simulink model "SP_CV3S"  (R2025b)
settings: Solver=VariableStepAuto  StartTime=0.0  StopTime=1200  RelTol=1e-3
values from neighbouring files (symbols this model uses):
  g = 9.81    [SP_CV3.m]
  mu = 0.62    [SP_CV3.m]
  Q10 = 0.01942    [SP_CV3.m]
  S1 = 1    [SP_CV3.m]
  S10 = 100 * 1e-4    (= 0.01)    [SP_CV3.m]
  S2 = 1    [SP_CV3.m]
  S20 = 100 * 1e-4    (= 0.01)    [SP_CV3.m]
settings Model: Creator=jakub  LastModifiedBy=jakub

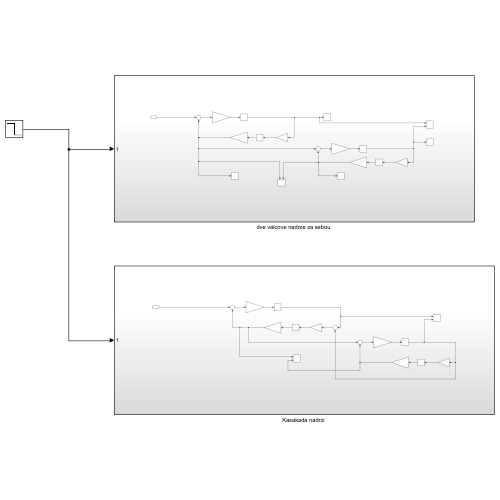
[thumbnail: Simulink's stored preview of the top-level diagram]
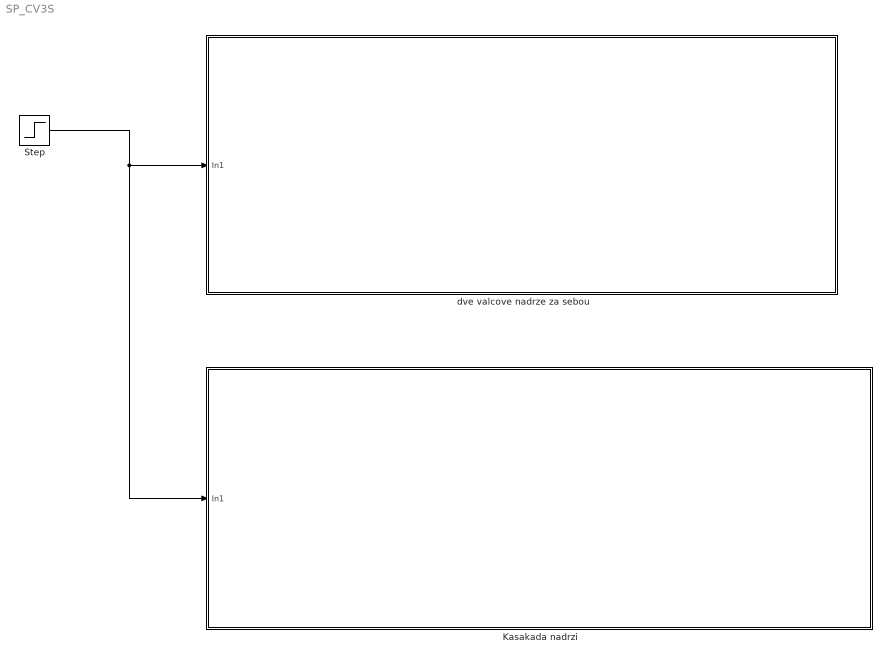
== system SP_CV3S ==
  "Kasakada nadrzi " : Subsystem
  Step : Step  Time=700  Before=Q10  After=Q10/2  SampleTime=0
  "dve valcove nadrze za sebou " : Subsystem
  wires:
  Step/1 -> "Kasakada nadrzi "/1(In1), "dve valcove nadrze za sebou "/1(In1)

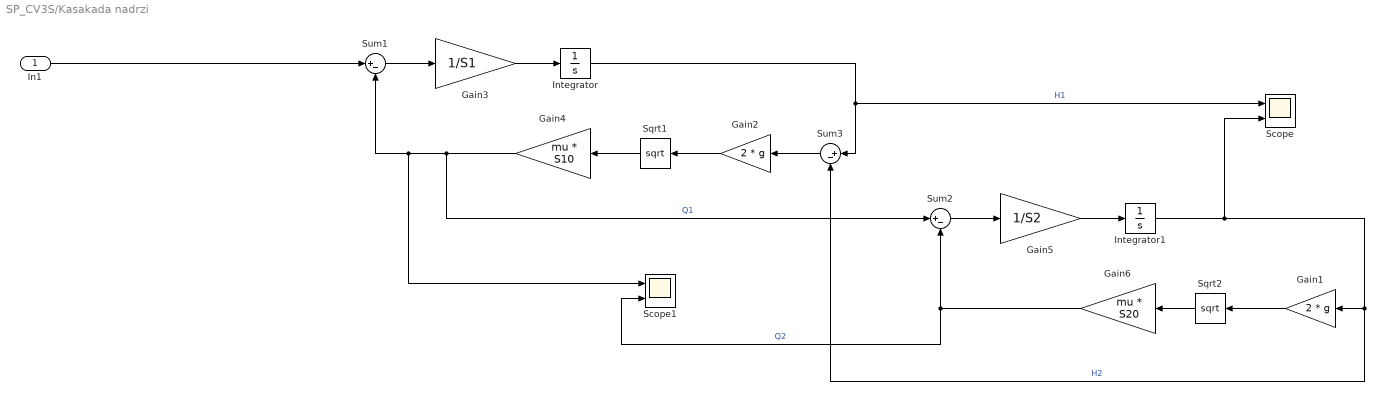
== system SP_CV3S/Kasakada nadrzi  ==
  In1 : Inport
  Gain1 : Gain  Gain=2 * g
  Gain2 : Gain  Gain=2 * g
  Gain3 : Gain  Gain=1/S1
  Gain4 : Gain  Gain=mu * S10
  Gain5 : Gain  Gain=1/S2
  Gain6 : Gain  Gain=mu * S20
  Integrator : Integrator
  Integrator1 : Integrator
  Scope : Scope  NumInputPorts=2
      settings: ActiveDisplayYMinimum=-0.12453477348635439  ActiveDisplayYMaximum=1.1208129613771898  DataLoggingVariableName=ScopeData6
  Scope1 : Scope  NumInputPorts=2
      settings: ActiveDisplayYMinimum=-0.0024239470723240262  ActiveDisplayYMaximum=0.021815523650916241  DataLoggingVariableName=ScopeData7
  Sqrt1 : Sqrt
  Sqrt2 : Sqrt
  Sum1 : Sum  Inputs=|+-
  Sum2 : Sum  Inputs=|+-
  Sum3 : Sum  Inputs=|+-
  wires:
  Integrator1/1 -> Scope/2, Sum3/2, Gain1/1  "H2"
  Gain6/1 -> Sum2/2, Scope1/2  "Q2"
  Gain3/1 -> Integrator/1
  Sqrt2/1 -> Gain6/1
  Gain4/1 -> Sum2/1, Scope1/1, Sum1/2  "Q1"
  Sum2/1 -> Gain5/1
  Integrator/1 -> Sum3/1, Scope/1  "H1"
  Gain2/1 -> Sqrt1/1
  In1/1 -> Sum1/1
  Gain5/1 -> Integrator1/1
  Gain1/1 -> Sqrt2/1
  Sum1/1 -> Gain3/1
  Sum3/1 -> Gain2/1
  Sqrt1/1 -> Gain4/1

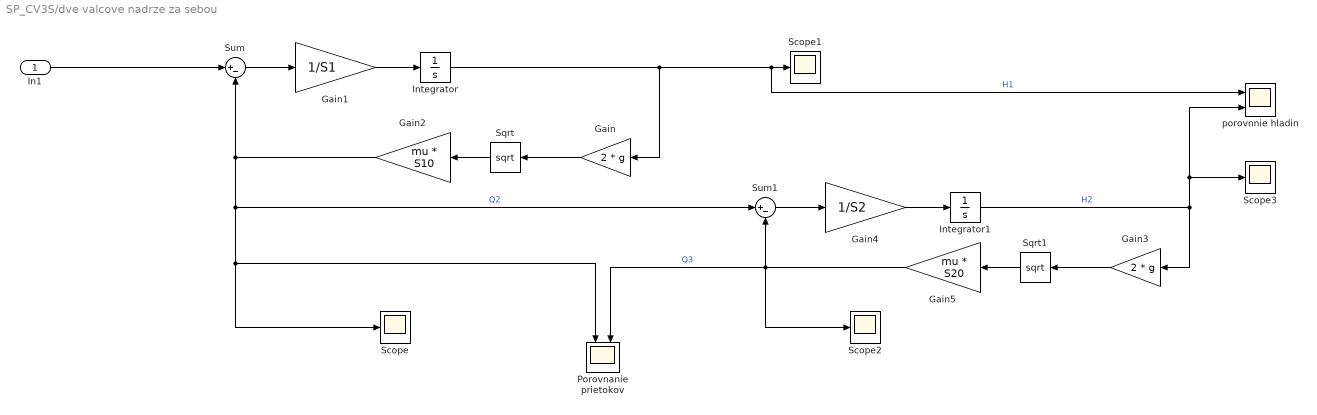
== system SP_CV3S/dve valcove nadrze za sebou  ==
  In1 : Inport
  Gain : Gain  Gain=2 * g
  Gain1 : Gain  Gain=1/S1
  Gain2 : Gain  Gain=mu * S10
  Gain3 : Gain  Gain=2 * g
  Gain4 : Gain  Gain=1/S2
  Gain5 : Gain  Gain=mu * S20
  Integrator : Integrator
  Integrator1 : Integrator
  "Porovnanie prietokov " : Scope  NumInputPorts=2
      settings: ActiveDisplayYMinimum=-0.011110072095082475  ActiveDisplayYMaximum=0.054945048812961729  DataLoggingVariableName=ScopeData4
  Scope{,1..3} (4 alike) : Scope
      Scope settings: ActiveDisplayYMinimum=-0.0050556906084998094  ActiveDisplayYMaximum=0.016018854700153219
      Scope1 settings: ActiveDisplayYMinimum=-0.32760461358028509  ActiveDisplayYMaximum=0.98489538641971508
      Scope2 settings: ActiveDisplayYMinimum=-0.021038308861334423  ActiveDisplayYMaximum=0.03767458597829737  DataLoggingVariableName=ScopeData2
      Scope3 settings: ActiveDisplayYMinimum=-0.32760461358028509  ActiveDisplayYMaximum=0.98489538641971508  DataLoggingVariableName=ScopeData3
  Sqrt : Sqrt
  Sqrt1 : Sqrt
  Sum : Sum  Inputs=|+-
  Sum1 : Sum  Inputs=|+-
  porovnnie hladin : Scope  NumInputPorts=2
      settings: ActiveDisplayYMinimum=-0.21250944448395515  ActiveDisplayYMaximum=3.2411920156842422  DataLoggingVariableName=ScopeData5
  wires:
  Integrator/1 -> Scope1/1, porovnnie hladin/1, Gain/1  "H1"
  Gain4/1 -> Integrator1/1
  Gain5/1 -> "Porovnanie prietokov "/2, Scope2/1, Sum1/2  "Q3"
  Gain2/1 -> "Porovnanie prietokov "/1, Scope/1, Sum1/1, Sum/2  "Q2"
  Sum/1 -> Gain1/1
  Gain/1 -> Sqrt/1
  Sqrt/1 -> Gain2/1
  Integrator1/1 -> porovnnie hladin/2, Scope3/1, Gain3/1  "H2"
  Sqrt1/1 -> Gain5/1
  Gain1/1 -> Integrator/1
  Sum1/1 -> Gain4/1
  Gain3/1 -> Sqrt1/1
  In1/1 -> Sum/1
